simulink model "TS_fuzzy_2017"  (R2017a)
settings: Solver=ode5  StartTime=0.0  StopTime=20  FixedStep=0.0005  RelTol=1e-3
model workspace (MAT data in the model file):
  A = {[0  1  0  0; 0  -0.02  4.71375609555  0.101638001338; 0  0  0  1; 0  0.02  -14.3808383038  -0.101638001338], [0  1  0  0; 0  -0.02  4.71375609555  -0.101638001338; 0  0  0  1; 0  0.02  -14.3808383038  0.101638001338], [0  1  0  0; 0  -0.02  4.71375609555  0.101638001338; 0  0  0  1; 0  0.0193185165258  -14.3808383038  -0.0981747704247], [0  1  0  0; 0  -0.02  4.71375609555  -0.101638001338; 0  0  0  1; 0  0.0193185165258  -14.3808383038  0.0981747704247], [0  1  0  0; 0  -0.0193518363836  4.71375609555  0.0983440986125; 0  0  0  1; 0  0.0193518363836  -14.3808383038  -0.0983440986125], [0  1  0  0; 0  -0.0193518363836  4.71375609555  -0.0983440986125; 0  0  0  1; 0  0.0193518363836  -14.3808383038  0.0983440986125], [0  1  0  0; 0  -0.0193518363836  4.71375609555  0.0983440986125; 0  0  0  1; 0  0.0186924385491  -14.3808383038  -0.0949931047129], [0  1  0  0; 0  -0.0193518363836  4.71375609555  -0.0983440986125; 0  0  0  1; 0  0.0186924385491  -14.3808383038  0.0949931047129]}
  B = {[0; 0.1; 0; -0.1], [0; 0.1; 0; -0.1], [0; 0.1; 0; -0.0965925826289], [0; 0.1; 0; -0.0965925826289], [0; 0.0967591819181; 0; -0.0967591819181], [0; 0.0967591819181; 0; -0.0967591819181], [0; 0.0967591819181; 0; -0.0934621927453], [0; 0.0967591819181; 0; -0.0934621927453]}
  Con = []
  Gamma = []
  Gammaij = []
  Ha = [0  0; 1  0; 0  0; 0  1]
  Inu = [1  0; 0  1]
  K1 = [1798.87901112 1746.27842226 -3664.10314747 1048.80683327]
  K2 = [1795.98565777 1743.50646299 -3658.48325147 1044.99138612]
  K3 = [1703.98941453 1655.96680666 -3484.47999338 990.835296289]
  K4 = [1707.11802484 1658.95756649 -3490.49487661 990.681349598]
  K5 = [1856.85127929 1802.60289828 -3782.48828479 1082.48851424]
  K6 = [1854.17487491 1800.04538442 -3777.34932857 1078.85160784]
  K7 = [1763.11138711 1713.38136291 -3605.01221665 1025.22219928]
  K8 = [1766.06272093 1716.20592194 -3610.71480684 1025.01001836]
  M = 10
  N = {[], [], [], [], [], [], [], []}
  P = []
  P_sol = [0.0810855738195  0.0826310566822  -0.0216804280872  -0.0367847266173; 0.0826310566822  0.793234251916  -0.181526275783  -0.542807016393; -0.0216804280872  -0.181526275783  0.0853419913182  0.100423678027; -0.0367847266173  -0.542807016393  0.100423678027  0.578582965098]
  Sig = Simulink.Signal
  Sig.DataType = 'auto'
  Sig.Dimensions = -1
  Sig.DimensionsMode = 'auto'
  Sig.Complexity = 'auto'
  Sig.SampleTime = -1
  Sig.SamplingMode = 'auto'
  Wa = [0  0  0.0190044572  0; 0  0  -0.0108558171612  0]
  a_m = 0.0961991039907
  a_r = 0.00380089143999
  alpha = -5
  b_m = 0.0978288319985
  b_r = 0.00217116343224
  crit = 0
  dres = [1.44166146102e-14; 2.82912004272e-13; 2.82749911058e-13; 2.66211439542e-13; 2.66161897275e-13; 2.829523378e-13; 2.82948374424e-13; 2.65932288025e-13; 2.66152454393e-13; 1.57841345448e-14; 1.77952311777e-14; 1.78043671686e-14; 1.56997678523e-14; 1.58169153337e-14; 1.7745046355e-14; 1.77684748226e-14; 1.77863995005e-14; 1.77983242906e-14; 1.5805440054e-14; 1.58287552354e-14; 1.77131220027e-14; 1.77387798414e-14; 1.57518356609e-14; 1.78061500935e-14; 1.78033515575e-14; 1.56377242516e-14; 1.57143395222e-14; 1.78048267026e-14; 1.78058575895e-14; 1.57051768739e-14; 1.57547175203e-14; 1.57190629733e-14; 1.77988426658e-14; 1.78040422032e-14; 1.77891543813e-14; 1.77982159919e-14; 1.56661417044e-14]
  g = 9.8
  i = 7
  j = 8
  k = 2
  k1 = 0.2
  k2 = 49
  k3 = -0.2
  k4 = -147
  k5 = 5
  k6 = -5
  k7 = -1
  l = 1
  m = 5
  mu = 0.2
  nu = 1
  nx = 4
  options_sdp : struct (value not decoded)
  pass_x1 = 0.002
  pass_x2 = 0.01
  pass_x3 = 0.000523598775598
  pass_x4 = 0.00157079632679
  primal = [0.0359108151649; 0.628144408932; 0.629129861861; 0.616150224715; 0.615982168518; 0.626707829845; 0.624695741632; 0.615928428678; 0.616069732322; 1.25754206722; 1.25334332917; 1.25620749446; 1.24522472918; 1.25197792492; 1.23225135193; 1.24307074086; 1.25386974908; 1.25667256078; 1.24021948895; 1.24815005943; 1.21895205647; 1.23063555901; 1.23220493884; 1.24976439964; 1.25207389268; 1.23150420655; 1.23205384648; 1.24622339792; 1.24908795247; 1.23134348304; 1.23217886304; 1.25165017164; 1.2551053183; 1.25403431724; 1.25004862946; 1.24846317584; 1.23200191607]
  solpb.yalmipversion = '20210331'
  solpb.matlabversion = '9.9.0.1467703 (R2020b)'
  solpb.yalmiptime = 0.3728979
  solpb.solvertime = 0.4961021
  solpb.info = 'Successfully solved (SeDuMi-1.3)'
  solpb.problem = 0
  taura = []
  x1_max = 2
  x1_min = 0
  x2_max = 5
  x2_min = -5
  x3 = 0.261799387799
  x3_max = 0.261799387799
  x3_min = -0.261799387799
  x4 = 0.785398163397
  x4_max = 0.785398163397
  x4_min = -0.785398163397
  z1 = 0.0967591819181
  z1_max = 0.1
  z1_min = 0.0967591819181
  z1s = [0.1 0.0967591819181]
  z2 = 0.965925826289
  z2_max = 1
  z2_min = 0.965925826289
  z2s = [1 0.965925826289]
  z3 = 0
  z3_max = 0.999999954307
  z3_min = 0.988615929465
  z3s = [0.999999954307 0.988615929465]
  z4 = -0.203276002676
  z4_max = 0.203276002676
  z4_min = -0.203276002676
  z4s = [0.203276002676 -0.203276002676]
settings Model: ParameterArgumentNames=K1,K2,K3,K4,K5,K6,K7,K8  OrderedModelArguments=off  Creator=Dell Precision  LastModifiedBy=Dell Precision
settings DataIOCC: ReturnWorkspaceOutputs=on
settings SFSimCC: SimUseLocalCustomCode=on
settings RTWCC: RTWUseLocalCustomCode=on

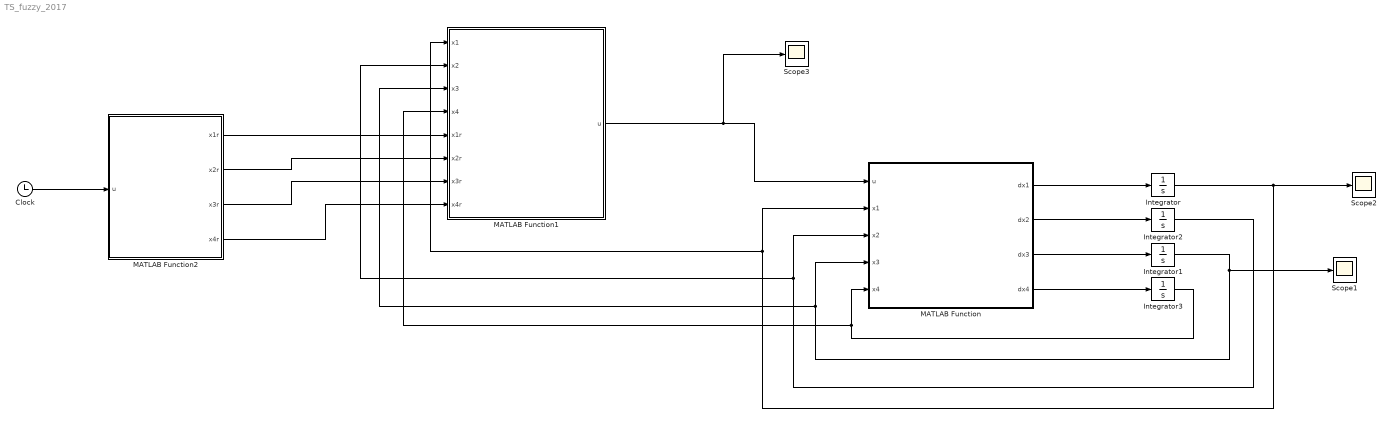
== system TS_fuzzy_2017 ==
  Clock : Clock
  Integrator : Integrator  InitialCondition=0.002
  Integrator1 : Integrator  InitialCondition=0.001
  Integrator2 : Integrator
  Integrator3 : Integrator
  MATLAB Function : MATLAB Function  TreatAsAtomicUnit=on
  MATLAB Function1 : MATLAB Function  TreatAsAtomicUnit=on
  MATLAB Function2 : MATLAB Function  TreatAsAtomicUnit=on
  Scope1 : Scope
  Scope2 : Scope
  Scope3 : Scope
  wires:
  MATLAB Function/1(dx1) -> Integrator/1
  MATLAB Function/3(dx3) -> Integrator1/1
  MATLAB Function/2(dx2) -> Integrator2/1
  MATLAB Function/4(dx4) -> Integrator3/1
  Integrator/1 -> Scope2/1, MATLAB Function1/1(x1), MATLAB Function/2(x1)
  Integrator2/1 -> MATLAB Function1/2(x2), MATLAB Function/3(x2)
  Integrator1/1 -> Scope1/1, MATLAB Function1/3(x3), MATLAB Function/4(x3)
  Integrator3/1 -> MATLAB Function1/4(x4), MATLAB Function/5(x4)
  MATLAB Function1/1(u) -> Scope3/1, MATLAB Function/1(u)
  MATLAB Function2/1(x1r) -> MATLAB Function1/5(x1r)
  MATLAB Function2/2(x2r) -> MATLAB Function1/6(x2r)
  MATLAB Function2/3(x3r) -> MATLAB Function1/7(x3r)
  MATLAB Function2/4(x4r) -> MATLAB Function1/8(x4r)
  Clock/1 -> MATLAB Function2/1(u)

== matlab function TS_fuzzy_2017/MATLAB Function1 ==
  data: x1 input; u output; x2 input; x3 input; x4 input; x1r input; x2r input; x3r input; x4r input
function u = controller(x1,x2,x3,x4,x1r,x2r,x3r,x4r)
M = 10;m=5;l=1;g=9.8;mu=0.2;
 z1_max = 1.0 ; z1_min =  0.096759181918094;
 z2_max = 1.0 ; z2_min = 0.965925826289068;
 z3_max = 1.0 ; z3_min = 0.988615929465369;
 z4_max = 0.203276002675801; z4_min = -0.203276002675801;
 
 z1 = 1/(M+m*sin(x3)^2);
 z2 = cos(x3);
 z3 = sin(x3)/x3;
 z4 = sin(x3)*x4;
 
 fx1_max = (z1 - z1_max)/(z1_max - z1_min);
 fx1_min = 1 - fx1_max;
 fx2_max = (z2 - z2_max)/(z2_max - z2_min);
 fx2_min = 1 - fx2_max;
 fx4_max = (z4 - z4_max)/(z4_max - z4_min);
 fx4_min = 1 - fx4_max;
 
 fx1 = [fx1_max;fx1_min];fx2 = [fx2_max;fx2_min];
 fx4 = [fx4_max;fx4_min];
 w = zeros(1,8);
 for i=1:1:2
     for j =1:1:2
         for k=1:1:2
             w(k+2*(j-1)+4*(i-1)) = fx1(i)*fx2(j)+fx4(k);
         end
     end
 end
 K1 = [12.573015167863607,11.670443174663127,21.647083956594344,-10.375610218596657];
 K2 = [12.561852981834190,11.640135437790097,21.667266506193606,-12.461324896105795];
 K3 = [12.579373722130569,11.330107265927644,22.592531362886690,-10.738986012330004];
 K4 = [12.585838671206071,11.346757367891286,22.587765778711585,-12.772521033036430];
 K5 = [12.986008214979357,12.023812191489590,22.438146547617315,-10.785917806786124];
 K6 = [12.978356581901147,12.005448868322016,22.455118060103267,-12.816147927103831];
 K7 = [12.983533861015832,11.672945666797634,23.387669783718934,-11.136074134801719];
 K8 = [13.005935842897038,11.719186355370148,23.339063489291300,-13.127111156361822];
 
%  K1 = [1.798879011121664e+03,1.746278422259811e+03,-3.664103147466416e+03,1.048806833265260e+03];
%  K2 = [1.795985657773947e+03,1.743506462990723e+03,-3.658483251474849e+03,1.044991386118453e+03];
%  K3 = [1.703989414532277e+03,1.655966806657551e+03,-3.484479993377050e+03,9.908352962892459e+02];
%  K4 = [1.707118024836941e+03,1.658957566491031e+03,-3.490494876605568e+03,9.906813495983950e+02];
%  K5 = [1.856851279294956e+03,1.802602898275560e+03,-3.782488284789967e+03,1.082488514238286e+03];
%  K6 = [1.854174874908221e+03,1.800045384419621e+03,-3.777349328565660e+03,1.078851607837832e+03];
%  K7 = [1.763111387109027e+03,1.713381362912869e+03,-3.605012216653592e+03,1.025222199284225e+03];
%  K8 = [1.766062720925707e+03,1.716205921942858e+03,-3.610714806836186e+03,1.025010018356801e+03];
 
 Kf = (w(1)*K1+w(2)*K2+w(3)*K3+w(4)*K4+w(5)*K5+w(6)*K6+w(7)*K7+w(8)*K8)/(w(1)+w(2)+w(3)+w(4)+w(5)+w(6)+w(7)+w(8));
 q = [x1;x2;x3;x4];
 qr = [x1r;x2r;x3r;x4r];
 u  = -Kf*(q-qr);

== matlab function TS_fuzzy_2017/MATLAB Function ==
  data: u input; dx1 output; x1 input; x2 input; x3 input; x4 input; dx2 output; dx3 output; dx4 output
function [dx1,dx2,dx3,dx4] = plant_model(u,x1,x2,x3,x4)
M = 10;m=5;l=1;g=9.8;mu=0.2;
q = [x1;x2;x3;x4];
a11 = -mu/(M+m*sin(x3)^2); a12 = m*g*cos(x3)*sin(x3)/((M+m*sin(x3)^2)*x3);
a13 = m*l*x4*sin(x3)/(M+m*sin(x3)^2); a21 = mu*cos(x3)/(l*(M+m*sin(x3)^2));
a22 = -(M+m)*g*sin(x3)/(l*x3*(M+m*sin(x3)^2)); a23=-m*x4*sin(x3)*cos(x3)/(M+m*sin(x3)^2);
b1 = 1/(M+m*sin(x3)^2); b2 = -cos(x3)/(l*(M+m*sin(x3)^2));
A = [0 1 0 0;0 a11 a12 a13;0 0 0 1;0 a21 a22 a23];
B = [0;b1;0;b2];

dq = A*q + B*u;
dx1 = dq(1);
dx2 = dq(2);
dx3 = dq(3);
dx4 = dq(4);

== matlab function TS_fuzzy_2017/MATLAB Function2 ==
  data: u input; x1r output; x2r output; x3r output; x4r output
function [x1r,x2r,x3r,x4r] = fcn(u)
 x1r = 0.6;
 x2r = 0;
 x3r = 0;
 x4r = 0;
